simulink model "pi_seqOfVariableSizeIface"  (R2018b)
settings: Solver=FixedStepDiscrete  StartTime=0.0  StopTime=10.0  RelTol=1e-3
undefined symbols (not defined in the file): arr, nCount
settings Model: Creator=matlab  LastModifiedBy=matlab
settings DataIOCC: SaveOutput=off  SignalLogging=off  SaveTime=off
settings OptimizationCC: DefaultParameterBehavior=Inlined  EnhancedBackFolding=on  PassReuseOutputArgsAs=Individual arguments  OptimizeBlockOrder=speed  DifferentSizesBufferReuse=on  OptimizationCustomize=off
settings DebuggingCC: ParameterTunabilityLossMsg=error
settings SFSimCC: MATLABDynamicMemAlloc=off
settings RTWCC: SystemTargetFile=ert.tlc  TemplateMakefile=ert_default_tmf  PostCodeGenCommand=packNGo(buildInfo);  GenerateReport=on  IncludeHyperlinkInReport=on  LaunchReport=on  GenerateTraceInfo=on  GenerateTraceReport=on  GenerateTraceReportSl=on  GenerateTraceReportSf=on  GenerateTraceReportEml=on
settings CodeAppCC: ForceParamTrailComments=on  IgnoreCustomStorageClasses=off  OperatorAnnotations=on  SimulinkDataObjDesc=on  SFDataObjDesc=on  InsertBlockDesc=on
settings ERTTargetCC: TargetLangStandard=C99 (ISO)  GenerateSampleERTMain=on  InlinedParameterPlacement=NonHierarchical  ERTCustomFileTemplate=example_file_process.tlc

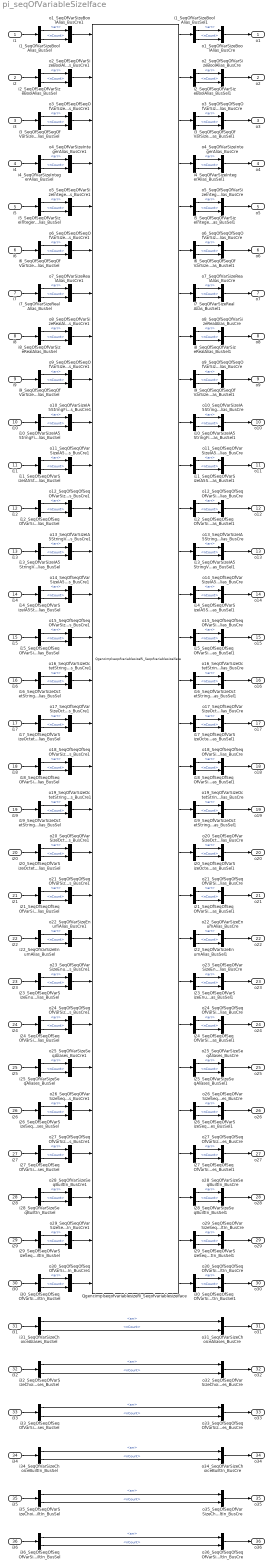
== system pi_seqOfVariableSizeIface ==
  i1 : Inport  OutDataTypeStr=Bus: SeqOfVarSizeBoolAlias  BusOutputAsStruct=on
  i2 : Inport  Port=2  OutDataTypeStr=Bus: SeqOfSeqOfVarSizeBoolAlias  BusOutputAsStruct=on
  i3 : Inport  Port=3  OutDataTypeStr=Bus: SeqOfSeqOfSeqOfVarSizeBoolAlias  BusOutputAsStruct=on
  i4 : Inport  Port=4  OutDataTypeStr=Bus: SeqOfVarSizeIntegerAlias  BusOutputAsStruct=on
  i5 : Inport  Port=5  OutDataTypeStr=Bus: SeqOfSeqOfVarSizeIntegerAlias  BusOutputAsStruct=on
  i6 : Inport  Port=6  OutDataTypeStr=Bus: SeqOfSeqOfSeqOfVarSizeIntegerAlias  BusOutputAsStruct=on
  i7 : Inport  Port=7  OutDataTypeStr=Bus: SeqOfVarSizeRealAlias  BusOutputAsStruct=on
  i8 : Inport  Port=8  OutDataTypeStr=Bus: SeqOfSeqOfVarSizeRealAlias  BusOutputAsStruct=on
  i9 : Inport  Port=9  OutDataTypeStr=Bus: SeqOfSeqOfSeqOfVarSizeRealAlias  BusOutputAsStruct=on
  i10 : Inport  Port=10  OutDataTypeStr=Bus: SeqOfVarSizeIA5StringFixedSizeAlias  BusOutputAsStruct=on
  i11 : Inport  Port=11  OutDataTypeStr=Bus: SeqOfSeqOfVarSizeIA5StringFixedSizeAlias  BusOutputAsStruct=on
  i12 : Inport  Port=12  OutDataTypeStr=Bus: SeqOfSeqOfSeqOfVarSizeIA5StringFixedSizeAlias  BusOutputAsStruct=on
  i13 : Inport  Port=13  OutDataTypeStr=Bus: SeqOfVarSizeIA5StringVarSizeAlias  BusOutputAsStruct=on
  i14 : Inport  Port=14  OutDataTypeStr=Bus: SeqOfSeqOfVarSizeIA5StringVarSizeAlias  BusOutputAsStruct=on
  i15 : Inport  Port=15  OutDataTypeStr=Bus: SeqOfSeqOfSeqOfVarSizeIA5StringVarSizeAlias  BusOutputAsStruct=on
  i16 : Inport  Port=16  OutDataTypeStr=Bus: SeqOfVarSizeOctetStringFixedSizeAlias  BusOutputAsStruct=on
  i17 : Inport  Port=17  OutDataTypeStr=Bus: SeqOfSeqOfVarSizeOctetStringFixedSizeAlias  BusOutputAsStruct=on
  i18 : Inport  Port=18  OutDataTypeStr=Bus: SeqOfSeqOfSeqOfVarSizeOctetStringFixedSizeAlias  BusOutputAsStruct=on
  i19 : Inport  Port=19  OutDataTypeStr=Bus: SeqOfVarSizeOctetStringVarSizeAlias  BusOutputAsStruct=on
  i20 : Inport  Port=20  OutDataTypeStr=Bus: SeqOfSeqOfVarSizeOctetStringVarSizeAlias  BusOutputAsStruct=on
  i21 : Inport  Port=21  OutDataTypeStr=Bus: SeqOfSeqOfSeqOfVarSizeOctetStringVarSizeAlias  BusOutputAsStruct=on
  i22 : Inport  Port=22  OutDataTypeStr=Bus: SeqOfVarSizeEnumAlias  BusOutputAsStruct=on
  i23 : Inport  Port=23  OutDataTypeStr=Bus: SeqOfSeqOfVarSizeEnumAlias  BusOutputAsStruct=on
  i24 : Inport  Port=24  OutDataTypeStr=Bus: SeqOfSeqOfSeqOfVarSizeEnumAlias  BusOutputAsStruct=on
  i25 : Inport  Port=25  OutDataTypeStr=Bus: SeqOfVarSizeSeqAliases  BusOutputAsStruct=on
  i26 : Inport  Port=26  OutDataTypeStr=Bus: SeqOfSeqOfVarSizeSeqAliases  BusOutputAsStruct=on
  i27 : Inport  Port=27  OutDataTypeStr=Bus: SeqOfSeqOfSeqOfVarSizeSeqAliases  BusOutputAsStruct=on
  i28 : Inport  Port=28  OutDataTypeStr=Bus: SeqOfVarSizeSeqBuiltIn  BusOutputAsStruct=on
  i29 : Inport  Port=29  OutDataTypeStr=Bus: SeqOfSeqOfVarSizeSeqBuiltIn  BusOutputAsStruct=on
  i30 : Inport  Port=30  OutDataTypeStr=Bus: SeqOfSeqOfSeqOfVarSizeSeqBuiltIn  BusOutputAsStruct=on
  i31 : Inport  Port=31  OutDataTypeStr=Bus: SeqOfVarSizeChoiceAliases  BusOutputAsStruct=on
  i32 : Inport  Port=32  OutDataTypeStr=Bus: SeqOfSeqOfVarSizeChoiceAliases  BusOutputAsStruct=on
  i33 : Inport  Port=33  OutDataTypeStr=Bus: SeqOfSeqOfSeqOfVarSizeChoiceAliases  BusOutputAsStruct=on
  i34 : Inport  Port=34  OutDataTypeStr=Bus: SeqOfVarSizeChoiceBuiltIn  BusOutputAsStruct=on
  i35 : Inport  Port=35  OutDataTypeStr=Bus: SeqOfSeqOfVarSizeChoiceBuiltIn  BusOutputAsStruct=on
  i36 : Inport  Port=36  OutDataTypeStr=Bus: SeqOfSeqOfSeqOfVarSizeChoiceBuiltIn  BusOutputAsStruct=on
  QgencimplseqofvariablesizeRi_Seqofvariablesizeiface : S-Function  FunctionName=QgencimplseqofvariablesizeRi_Seqofvariablesizeiface  SFunctionDeploymentMode=off  EnableBusSupport=off  mask(Legacy Function){SFunctionSpec=void qgencimplseqofvariablesize_RI_ri_seqOfVariableSizeIface(SeqOfVarSizeBoolAlias u1[1], SeqOfSeqOfVarSizeBoolAlias u2[1], SeqOfSeqOfSeqOfVarSizeBoolAlias u3[1], SeqOfVarSizeIntegerAlias u4[1], SeqOfSeqOfVarSizeIntegerAlias u5[1], SeqOfSeqOfSeqOfVarSizeIntegerAlias u6[1], SeqOfVarSizeRealAlias u7[1], SeqOfSeqOfVarSizeRealAlias u8[1], SeqOfSeqOfSeqOfVarSizeRealAlias u9[1], SeqOfVarSizeIA5StringFixedSizeAlias u10[1], SeqOfSeqOfVarSizeIA5StringFixedSizeAlias u11[1], SeqOfSeqOfSeqOfVarSizeIA5StringFixedSizeAlias u12[1], SeqOfVarSizeIA5StringVarSizeAlias u13[1], SeqOfSeqOfVarSizeIA5StringVarSizeAlias u14[1], SeqOfSeqOfSeqOfVarSizeIA5StringVarSizeAlias u15[1], SeqOfVarSizeOctetStringFixedSizeAlias u16[1], SeqOfSeqOfVarSizeOctetStringFixedSizeAlias u17[1], SeqOfSeqOfSeqOfVarSizeOctetStringFixedSizeAlias u18[1], SeqOfVarSizeOctetStringVarSizeAlias u19[1], SeqOfSeqOfVarSizeOctetStringVarSizeAlias u20[1], SeqOfSeqOfSeqOfVarSizeOctetStringVarSizeAlias u21[1], SeqOfVarSizeEnumAlias u22[1], SeqOfSeqOfVarSizeEnumAlias u23[1], SeqOfSeqOfSeqOfVarSizeEnumAlias u24[1], SeqOfVarSizeSeqAliases u25[1], SeqOfSeqOfVarSizeSeqAliases u26[1], SeqOfSeqOfSeqOfVarSizeSeqAliases u27[1], SeqOfVarSizeSeqBuiltIn u28[1], SeqOfSeqOfVarSizeSeqBuiltIn u29[1], SeqOfSeqOfSeqOfVarSizeSeqBuiltIn u30[1], SeqOfVarSizeBoolAlias y1[1], SeqOfSeqOfVarSizeBoolAlias y2[1], SeqOfSeqOfSeqOfVarSizeBoolAlias y3[1], SeqOfVarSizeIntegerAlias y4[1], SeqOfSeqOfVarSizeIntegerAlias y5[1], SeqOfSeqOfSeqOfVarSizeIntegerAlias y6[1], SeqOfVarSizeRealAlias y7[1], SeqOfSeqOfVarSizeRealAlias y8[1], SeqOfSeqOfSeqOfVarSizeRealAlias y9[1], SeqOfVarSizeIA5StringFixedSizeAlias y10[1], SeqOfSeqOfVarSizeIA5StringFixedSizeAlias y11[1], SeqOfSeqOfSeqOfVarSizeIA5StringFixedSizeAlias y12[1], SeqOfVarSizeIA5StringVarSizeAlias y13[1], SeqOfSeqOfVarSizeIA5StringVarSizeAlias y14[1], SeqOfSeqOfSeqOfVarSizeIA5StringVarSizeAlias y15[1], SeqOfVarSizeOctetStringFixedSizeAlias y16[1], SeqOfSeqOfVarSizeOctetStringFixedSizeAlias y17[1], SeqOfSeqOfSeqOfVarSizeOctetStringFixedSizeAlias y18[1], SeqOfVarSizeOctetStringVarSizeAlias y19[1], SeqOfSeqOfVarSizeOctetStringVarSizeAlias y20[1], SeqOfSeqOfSeqOfVarSizeOctetStringVarSizeAlias y21[1], SeqOfVarSizeEnumAlias y22[1], SeqOfSeqOfVarSizeEnumAlias y23[1], SeqOfSeqOfSeqOfVarSizeEnumAlias y24[1], SeqOfVarSizeSeqAliases y25[1], SeqOfSeqOfVarSizeSeqAliases y26[1], SeqOfSeqOfSeqOfVarSizeSeqAliases y27[1], SeqOfVarSizeSeqBuiltIn y28[1], SeqOfSeqOfVarSizeSeqBuiltIn y29[1], SeqOfSeqOfSeqOfVarSizeSeqBuiltIn y30[1]), ShowSpec=off}
      mask prompts: ShowSpec "Display function specification"
      mask help:
      | This block allows you to call the legacy functions specified by the following Legacy Code Tool definition:
      | def.SFunctionName = 'QgencimplseqofvariablesizeRi_Seqofvariablesizeiface';
      | def.OutputFcnSpec = 'void qgencimplseqofvariablesize_RI_ri_seqOfVariableSizeIface(SeqOfVarSizeBoolAlias u1[1], SeqOfSeqOfVarSizeBoolAlias u2[1], SeqOfSeqOfSeqOfVarSizeBoolAlias u3[1], SeqOfVarSizeIntegerAlias u4[1], SeqOfSeqOfVarSizeIntegerAlias u5[1], SeqOfSeqOfSeqOfVarSizeIntegerAlias u6[1], SeqOfVarSizeRealAlias u7[1], SeqOfSeqOfVarSizeRealAlias u8[1], SeqOfSeqOfSeqOfVarSizeRealAlias u9[1], SeqOfVarSizeIA5StringFixedSizeAlias u10[1], SeqOfSeqOfVarSizeIA5StringFixedSizeAlias u11[1], SeqOfSeqOfSeqOfVarSizeIA5StringFixedSizeAlias u12[1], SeqOfVarSizeIA5StringVarSizeAlias u13[1], SeqOfSeqOfVarSizeIA5StringVarSizeAlias u14[1], SeqOfSeqOfSeqOfVarSizeIA5StringVarSizeAlias u15[1], SeqOfVarSizeOctetStringFixedSizeAlias u16[1], SeqOfSeqOfVarSizeOctetStringFixedSizeAlias u17[1], SeqOfSeqOfSeqOfVarSizeOctetStringFixedSizeAlias u18[1], SeqOfVarSizeOctetStringVarSizeAlias u19[1], SeqOfSeqOfVarSizeOctetStringVarSizeAlias u20[1], SeqOfSeqOfSeqOfVarSizeOctetStringVarSizeAlias u21[1], SeqOfVarSizeEnumAlias u22[1], SeqOfSeqOfVarSizeEnumAlias u23[1], SeqOfSeqOfSeqOfVarSizeEnumAlias u24[1], SeqOfVarSizeSeqAliases u25[1], SeqOfSeqOfVarSizeSeqAliases u26[1], SeqOfSeqOfSeqOfVarSizeSeqAliases u27[1], SeqOfVarSizeSeqBuiltIn u28[1], SeqOfSeqOfVarSizeSeqBuiltIn u29[1], SeqOfSeqOfSeqOfVarSizeSeqBuiltIn u30[1], SeqOfVarSizeBoolAlias y1[1], SeqOfSeqOfVarSizeBoolAlias y2[1], SeqOfSeqOfSeqOfVarSizeBoolAlias y3[1], SeqOfVarSizeIntegerAlias y4[1], SeqOfSeqOfVarSizeIntegerAlias y5[1], SeqOfSeqOfSeqOfVarSizeIntegerAlias y6[1], SeqOfVarSizeRealAlias y7[1], SeqOfSeqOfVarSizeRealAlias y8[1], SeqOfSeqOfSeqOfVarSizeRealAlias y9[1], SeqOfVarSizeIA5StringFixedSizeAlias y10[1], SeqOfSeqOfVarSizeIA5StringFixedSizeAlias y11[1], SeqOfSeqOfSeqOfVarSizeIA5StringFixedSizeAlias y12[1], SeqOfVarSizeIA5StringVarSizeAlias y13[1], SeqOfSeqOfVarSizeIA5StringVarSizeAlias y14[1], SeqOfSeqOfSeqOfVarSizeIA5StringVarSizeAlias y15[1], SeqOfVarSizeOctetStringFixedSizeAlias y16[1], SeqOfSeqOfVarSizeOctetStringFixedSizeAlias y17[1], SeqOfSeqOfSeqOfVarSizeOctetStringFixedSizeAlias y18[1], SeqOfVarSizeOctetStringVarSizeAlias y19[1], SeqOfSeqOfVarSizeOctetStringVarSizeAlias y20[1], SeqOfSeqOfSeqOfVarSizeOctetStringVarSizeAlias y21[1], SeqOfVarSizeEnumAlias y22[1], SeqOfSeqOfVarSizeEnumAlias y23[1], SeqOfSeqOfSeqOfVarSizeEnumAlias y24[1], SeqOfVarSizeSeqAliases y25[1], SeqOfSeqOfVarSizeSeqAliases y26[1], SeqOfSeqOfSeqOfVarSizeSeqAliases y27[1], SeqOfVarSizeSeqBuiltIn y28[1], SeqOfSeqOfVarSizeSeqBuiltIn y29[1], SeqOfSeqOfSeqOfVarSizeSeqBuiltIn y30[1])';
      | def.HeaderFiles = {'qgencimplseqofvariablesize_invoke_ri.h'};
      | def.SourceFiles = {'qgencimplseqofvariablesize_invoke_ri.c'};
      | def.IncPaths = {'..\..\..\dataview\C'};
      mask Help: <p>This block was generated automatically by the Legacy Code Tool. For detailed help on this tool, call<a href="matlab:legacy_code('help')"> legacy_code('help')</a>.</p>
      mask Callback ShowSpec:
      | if strcmp(get_param(gcbh, 'ShowSpec'), 'on')
      |   set_param(gcbh, 'MaskDisplay', sprintf('fprintf(''%s'');', get_param(gcbh, 'SFunctionSpec')));
      | else
      |   set_param(gcbh, 'MaskDisplay', sprintf('fprintf(''%s'');', get_param(gcbh, 'FunctionName')));
      | end
      mask Display: fprintf('QgencimplseqofvariablesizeRi_Seqofvariablesizeiface');
  i10_SeqOfVarSizeIA5StringFixedSizeAlias_BusSel : BusSelector  OutputSignals=arr,nCount
  i10_SeqOfVarSizeIA5StringFixedSizeAlias_BusSel1 : BusSelector  OutputSignals=arr,nCount
  i11_SeqOfSeqOfVarSizeIA5StringFixedSizeAlias_BusSel : BusSelector  OutputSignals=arr,nCount
  i11_SeqOfSeqOfVarSizeIA5StringFixedSizeAlias_BusSel1 : BusSelector  OutputSignals=arr,nCount
  i12_SeqOfSeqOfSeqOfVarSizeIA5StringFixedSizeAlias_BusSel : BusSelector  OutputSignals=arr,nCount
  i12_SeqOfSeqOfSeqOfVarSizeIA5StringFixedSizeAlias_BusSel1 : BusSelector  OutputSignals=arr,nCount
  i13_SeqOfVarSizeIA5StringVarSizeAlias_BusSel : BusSelector  OutputSignals=arr,nCount
  i13_SeqOfVarSizeIA5StringVarSizeAlias_BusSel1 : BusSelector  OutputSignals=arr,nCount
  i14_SeqOfSeqOfVarSizeIA5StringVarSizeAlias_BusSel : BusSelector  OutputSignals=arr,nCount
  i14_SeqOfSeqOfVarSizeIA5StringVarSizeAlias_BusSel1 : BusSelector  OutputSignals=arr,nCount
  i15_SeqOfSeqOfSeqOfVarSizeIA5StringVarSizeAlias_BusSel : BusSelector  OutputSignals=arr,nCount
  i15_SeqOfSeqOfSeqOfVarSizeIA5StringVarSizeAlias_BusSel1 : BusSelector  OutputSignals=arr,nCount
  i16_SeqOfVarSizeOctetStringFixedSizeAlias_BusSel : BusSelector  OutputSignals=arr,nCount
  i16_SeqOfVarSizeOctetStringFixedSizeAlias_BusSel1 : BusSelector  OutputSignals=arr,nCount
  i17_SeqOfSeqOfVarSizeOctetStringFixedSizeAlias_BusSel : BusSelector  OutputSignals=arr,nCount
  i17_SeqOfSeqOfVarSizeOctetStringFixedSizeAlias_BusSel1 : BusSelector  OutputSignals=arr,nCount
  i18_SeqOfSeqOfSeqOfVarSizeOctetStringFixedSizeAlias_BusSel : BusSelector  OutputSignals=arr,nCount
  i18_SeqOfSeqOfSeqOfVarSizeOctetStringFixedSizeAlias_BusSel1 : BusSelector  OutputSignals=arr,nCount
  i19_SeqOfVarSizeOctetStringVarSizeAlias_BusSel : BusSelector  OutputSignals=arr,nCount
  i19_SeqOfVarSizeOctetStringVarSizeAlias_BusSel1 : BusSelector  OutputSignals=arr,nCount
  i1_SeqOfVarSizeBoolAlias_BusSel : BusSelector  OutputSignals=arr,nCount
  i1_SeqOfVarSizeBoolAlias_BusSel1 : BusSelector  OutputSignals=arr,nCount
  i20_SeqOfSeqOfVarSizeOctetStringVarSizeAlias_BusSel : BusSelector  OutputSignals=arr,nCount
  i20_SeqOfSeqOfVarSizeOctetStringVarSizeAlias_BusSel1 : BusSelector  OutputSignals=arr,nCount
  i21_SeqOfSeqOfSeqOfVarSizeOctetStringVarSizeAlias_BusSel : BusSelector  OutputSignals=arr,nCount
  i21_SeqOfSeqOfSeqOfVarSizeOctetStringVarSizeAlias_BusSel1 : BusSelector  OutputSignals=arr,nCount
  i22_SeqOfVarSizeEnumAlias_BusSel : BusSelector  OutputSignals=arr,nCount
  i22_SeqOfVarSizeEnumAlias_BusSel1 : BusSelector  OutputSignals=arr,nCount
  i23_SeqOfSeqOfVarSizeEnumAlias_BusSel : BusSelector  OutputSignals=arr,nCount
  i23_SeqOfSeqOfVarSizeEnumAlias_BusSel1 : BusSelector  OutputSignals=arr,nCount
  i24_SeqOfSeqOfSeqOfVarSizeEnumAlias_BusSel : BusSelector  OutputSignals=arr,nCount
  i24_SeqOfSeqOfSeqOfVarSizeEnumAlias_BusSel1 : BusSelector  OutputSignals=arr,nCount
  i25_SeqOfVarSizeSeqAliases_BusSel : BusSelector  OutputSignals=arr,nCount
  i25_SeqOfVarSizeSeqAliases_BusSel1 : BusSelector  OutputSignals=arr,nCount
  i26_SeqOfSeqOfVarSizeSeqAliases_BusSel : BusSelector  OutputSignals=arr,nCount
  i26_SeqOfSeqOfVarSizeSeqAliases_BusSel1 : BusSelector  OutputSignals=arr,nCount
  i27_SeqOfSeqOfSeqOfVarSizeSeqAliases_BusSel : BusSelector  OutputSignals=arr,nCount
  i27_SeqOfSeqOfSeqOfVarSizeSeqAliases_BusSel1 : BusSelector  OutputSignals=arr,nCount
  i28_SeqOfVarSizeSeqBuiltIn_BusSel : BusSelector  OutputSignals=arr,nCount
  i28_SeqOfVarSizeSeqBuiltIn_BusSel1 : BusSelector  OutputSignals=arr,nCount
  i29_SeqOfSeqOfVarSizeSeqBuiltIn_BusSel : BusSelector  OutputSignals=arr,nCount
  i29_SeqOfSeqOfVarSizeSeqBuiltIn_BusSel1 : BusSelector  OutputSignals=arr,nCount
  i2_SeqOfSeqOfVarSizeBoolAlias_BusSel : BusSelector  OutputSignals=arr,nCount
  i2_SeqOfSeqOfVarSizeBoolAlias_BusSel1 : BusSelector  OutputSignals=arr,nCount
  i30_SeqOfSeqOfSeqOfVarSizeSeqBuiltIn_BusSel : BusSelector  OutputSignals=arr,nCount
  i30_SeqOfSeqOfSeqOfVarSizeSeqBuiltIn_BusSel1 : BusSelector  OutputSignals=arr,nCount
  i31_SeqOfVarSizeChoiceAliases_BusSel : BusSelector  OutputSignals=arr,nCount
  i32_SeqOfSeqOfVarSizeChoiceAliases_BusSel : BusSelector  OutputSignals=arr,nCount
  i33_SeqOfSeqOfSeqOfVarSizeChoiceAliases_BusSel : BusSelector  OutputSignals=arr,nCount
  i34_SeqOfVarSizeChoiceBuiltIn_BusSel : BusSelector  OutputSignals=arr,nCount
  i35_SeqOfSeqOfVarSizeChoiceBuiltIn_BusSel : BusSelector  OutputSignals=arr,nCount
  i36_SeqOfSeqOfSeqOfVarSizeChoiceBuiltIn_BusSel : BusSelector  OutputSignals=arr,nCount
  i3_SeqOfSeqOfSeqOfVarSizeBoolAlias_BusSel : BusSelector  OutputSignals=arr,nCount
  i3_SeqOfSeqOfSeqOfVarSizeBoolAlias_BusSel1 : BusSelector  OutputSignals=arr,nCount
  i4_SeqOfVarSizeIntegerAlias_BusSel : BusSelector  OutputSignals=arr,nCount
  i4_SeqOfVarSizeIntegerAlias_BusSel1 : BusSelector  OutputSignals=arr,nCount
  i5_SeqOfSeqOfVarSizeIntegerAlias_BusSel : BusSelector  OutputSignals=arr,nCount
  i5_SeqOfSeqOfVarSizeIntegerAlias_BusSel1 : BusSelector  OutputSignals=arr,nCount
  i6_SeqOfSeqOfSeqOfVarSizeIntegerAlias_BusSel : BusSelector  OutputSignals=arr,nCount
  i6_SeqOfSeqOfSeqOfVarSizeIntegerAlias_BusSel1 : BusSelector  OutputSignals=arr,nCount
  i7_SeqOfVarSizeRealAlias_BusSel : BusSelector  OutputSignals=arr,nCount
  i7_SeqOfVarSizeRealAlias_BusSel1 : BusSelector  OutputSignals=arr,nCount
  i8_SeqOfSeqOfVarSizeRealAlias_BusSel : BusSelector  OutputSignals=arr,nCount
  i8_SeqOfSeqOfVarSizeRealAlias_BusSel1 : BusSelector  OutputSignals=arr,nCount
  i9_SeqOfSeqOfSeqOfVarSizeRealAlias_BusSel : BusSelector  OutputSignals=arr,nCount
  i9_SeqOfSeqOfSeqOfVarSizeRealAlias_BusSel1 : BusSelector  OutputSignals=arr,nCount
  o10_SeqOfVarSizeIA5StringFixedSizeAlias_BusCre : BusCreator  Inputs=arr,nCount  OutDataTypeStr=Bus: SeqOfVarSizeIA5StringFixedSizeAlias  NonVirtualBus=on
  o10_SeqOfVarSizeIA5StringFixedSizeAlias_BusCre1 : BusCreator  Inputs=arr,nCount  OutDataTypeStr=Bus: SeqOfVarSizeIA5StringFixedSizeAlias  NonVirtualBus=on
  o11_SeqOfSeqOfVarSizeIA5StringFixedSizeAlias_BusCre : BusCreator  Inputs=arr,nCount  OutDataTypeStr=Bus: SeqOfSeqOfVarSizeIA5StringFixedSizeAlias  NonVirtualBus=on
  o11_SeqOfSeqOfVarSizeIA5StringFixedSizeAlias_BusCre1 : BusCreator  Inputs=arr,nCount  OutDataTypeStr=Bus: SeqOfSeqOfVarSizeIA5StringFixedSizeAlias  NonVirtualBus=on
  o12_SeqOfSeqOfSeqOfVarSizeIA5StringFixedSizeAlias_BusCre : BusCreator  Inputs=arr,nCount  OutDataTypeStr=Bus: SeqOfSeqOfSeqOfVarSizeIA5StringFixedSizeAlias  NonVirtualBus=on
  o12_SeqOfSeqOfSeqOfVarSizeIA5StringFixedSizeAlias_BusCre1 : BusCreator  Inputs=arr,nCount  OutDataTypeStr=Bus: SeqOfSeqOfSeqOfVarSizeIA5StringFixedSizeAlias  NonVirtualBus=on
  o13_SeqOfVarSizeIA5StringVarSizeAlias_BusCre : BusCreator  Inputs=arr,nCount  OutDataTypeStr=Bus: SeqOfVarSizeIA5StringVarSizeAlias  NonVirtualBus=on
  o13_SeqOfVarSizeIA5StringVarSizeAlias_BusCre1 : BusCreator  Inputs=arr,nCount  OutDataTypeStr=Bus: SeqOfVarSizeIA5StringVarSizeAlias  NonVirtualBus=on
  o14_SeqOfSeqOfVarSizeIA5StringVarSizeAlias_BusCre : BusCreator  Inputs=arr,nCount  OutDataTypeStr=Bus: SeqOfSeqOfVarSizeIA5StringVarSizeAlias  NonVirtualBus=on
  o14_SeqOfSeqOfVarSizeIA5StringVarSizeAlias_BusCre1 : BusCreator  Inputs=arr,nCount  OutDataTypeStr=Bus: SeqOfSeqOfVarSizeIA5StringVarSizeAlias  NonVirtualBus=on
  o15_SeqOfSeqOfSeqOfVarSizeIA5StringVarSizeAlias_BusCre : BusCreator  Inputs=arr,nCount  OutDataTypeStr=Bus: SeqOfSeqOfSeqOfVarSizeIA5StringVarSizeAlias  NonVirtualBus=on
  o15_SeqOfSeqOfSeqOfVarSizeIA5StringVarSizeAlias_BusCre1 : BusCreator  Inputs=arr,nCount  OutDataTypeStr=Bus: SeqOfSeqOfSeqOfVarSizeIA5StringVarSizeAlias  NonVirtualBus=on
  o16_SeqOfVarSizeOctetStringFixedSizeAlias_BusCre : BusCreator  Inputs=arr,nCount  OutDataTypeStr=Bus: SeqOfVarSizeOctetStringFixedSizeAlias  NonVirtualBus=on
  o16_SeqOfVarSizeOctetStringFixedSizeAlias_BusCre1 : BusCreator  Inputs=arr,nCount  OutDataTypeStr=Bus: SeqOfVarSizeOctetStringFixedSizeAlias  NonVirtualBus=on
  o17_SeqOfSeqOfVarSizeOctetStringFixedSizeAlias_BusCre : BusCreator  Inputs=arr,nCount  OutDataTypeStr=Bus: SeqOfSeqOfVarSizeOctetStringFixedSizeAlias  NonVirtualBus=on
  o17_SeqOfSeqOfVarSizeOctetStringFixedSizeAlias_BusCre1 : BusCreator  Inputs=arr,nCount  OutDataTypeStr=Bus: SeqOfSeqOfVarSizeOctetStringFixedSizeAlias  NonVirtualBus=on
  o18_SeqOfSeqOfSeqOfVarSizeOctetStringFixedSizeAlias_BusCre : BusCreator  Inputs=arr,nCount  OutDataTypeStr=Bus: SeqOfSeqOfSeqOfVarSizeOctetStringFixedSizeAlias  NonVirtualBus=on
  o18_SeqOfSeqOfSeqOfVarSizeOctetStringFixedSizeAlias_BusCre1 : BusCreator  Inputs=arr,nCount  OutDataTypeStr=Bus: SeqOfSeqOfSeqOfVarSizeOctetStringFixedSizeAlias  NonVirtualBus=on
  o19_SeqOfVarSizeOctetStringVarSizeAlias_BusCre : BusCreator  Inputs=arr,nCount  OutDataTypeStr=Bus: SeqOfVarSizeOctetStringVarSizeAlias  NonVirtualBus=on
  o19_SeqOfVarSizeOctetStringVarSizeAlias_BusCre1 : BusCreator  Inputs=arr,nCount  OutDataTypeStr=Bus: SeqOfVarSizeOctetStringVarSizeAlias  NonVirtualBus=on
  o1_SeqOfVarSizeBoolAlias_BusCre : BusCreator  Inputs=arr,nCount  OutDataTypeStr=Bus: SeqOfVarSizeBoolAlias  NonVirtualBus=on
  o1_SeqOfVarSizeBoolAlias_BusCre1 : BusCreator  Inputs=arr,nCount  OutDataTypeStr=Bus: SeqOfVarSizeBoolAlias  NonVirtualBus=on
  o20_SeqOfSeqOfVarSizeOctetStringVarSizeAlias_BusCre : BusCreator  Inputs=arr,nCount  OutDataTypeStr=Bus: SeqOfSeqOfVarSizeOctetStringVarSizeAlias  NonVirtualBus=on
  o20_SeqOfSeqOfVarSizeOctetStringVarSizeAlias_BusCre1 : BusCreator  Inputs=arr,nCount  OutDataTypeStr=Bus: SeqOfSeqOfVarSizeOctetStringVarSizeAlias  NonVirtualBus=on
  o21_SeqOfSeqOfSeqOfVarSizeOctetStringVarSizeAlias_BusCre : BusCreator  Inputs=arr,nCount  OutDataTypeStr=Bus: SeqOfSeqOfSeqOfVarSizeOctetStringVarSizeAlias  NonVirtualBus=on
  o21_SeqOfSeqOfSeqOfVarSizeOctetStringVarSizeAlias_BusCre1 : BusCreator  Inputs=arr,nCount  OutDataTypeStr=Bus: SeqOfSeqOfSeqOfVarSizeOctetStringVarSizeAlias  NonVirtualBus=on
  o22_SeqOfVarSizeEnumAlias_BusCre : BusCreator  Inputs=arr,nCount  OutDataTypeStr=Bus: SeqOfVarSizeEnumAlias  NonVirtualBus=on
  o22_SeqOfVarSizeEnumAlias_BusCre1 : BusCreator  Inputs=arr,nCount  OutDataTypeStr=Bus: SeqOfVarSizeEnumAlias  NonVirtualBus=on
  o23_SeqOfSeqOfVarSizeEnumAlias_BusCre : BusCreator  Inputs=arr,nCount  OutDataTypeStr=Bus: SeqOfSeqOfVarSizeEnumAlias  NonVirtualBus=on
  o23_SeqOfSeqOfVarSizeEnumAlias_BusCre1 : BusCreator  Inputs=arr,nCount  OutDataTypeStr=Bus: SeqOfSeqOfVarSizeEnumAlias  NonVirtualBus=on
  o24_SeqOfSeqOfSeqOfVarSizeEnumAlias_BusCre : BusCreator  Inputs=arr,nCount  OutDataTypeStr=Bus: SeqOfSeqOfSeqOfVarSizeEnumAlias  NonVirtualBus=on
  o24_SeqOfSeqOfSeqOfVarSizeEnumAlias_BusCre1 : BusCreator  Inputs=arr,nCount  OutDataTypeStr=Bus: SeqOfSeqOfSeqOfVarSizeEnumAlias  NonVirtualBus=on
  o25_SeqOfVarSizeSeqAliases_BusCre : BusCreator  Inputs=arr,nCount  OutDataTypeStr=Bus: SeqOfVarSizeSeqAliases  NonVirtualBus=on
  o25_SeqOfVarSizeSeqAliases_BusCre1 : BusCreator  Inputs=arr,nCount  OutDataTypeStr=Bus: SeqOfVarSizeSeqAliases  NonVirtualBus=on
  o26_SeqOfSeqOfVarSizeSeqAliases_BusCre : BusCreator  Inputs=arr,nCount  OutDataTypeStr=Bus: SeqOfSeqOfVarSizeSeqAliases  NonVirtualBus=on
  o26_SeqOfSeqOfVarSizeSeqAliases_BusCre1 : BusCreator  Inputs=arr,nCount  OutDataTypeStr=Bus: SeqOfSeqOfVarSizeSeqAliases  NonVirtualBus=on
  o27_SeqOfSeqOfSeqOfVarSizeSeqAliases_BusCre : BusCreator  Inputs=arr,nCount  OutDataTypeStr=Bus: SeqOfSeqOfSeqOfVarSizeSeqAliases  NonVirtualBus=on
  o27_SeqOfSeqOfSeqOfVarSizeSeqAliases_BusCre1 : BusCreator  Inputs=arr,nCount  OutDataTypeStr=Bus: SeqOfSeqOfSeqOfVarSizeSeqAliases  NonVirtualBus=on
  o28_SeqOfVarSizeSeqBuiltIn_BusCre : BusCreator  Inputs=arr,nCount  OutDataTypeStr=Bus: SeqOfVarSizeSeqBuiltIn  NonVirtualBus=on
  o28_SeqOfVarSizeSeqBuiltIn_BusCre1 : BusCreator  Inputs=arr,nCount  OutDataTypeStr=Bus: SeqOfVarSizeSeqBuiltIn  NonVirtualBus=on
  o29_SeqOfSeqOfVarSizeSeqBuiltIn_BusCre : BusCreator  Inputs=arr,nCount  OutDataTypeStr=Bus: SeqOfSeqOfVarSizeSeqBuiltIn  NonVirtualBus=on
  o29_SeqOfSeqOfVarSizeSeqBuiltIn_BusCre1 : BusCreator  Inputs=arr,nCount  OutDataTypeStr=Bus: SeqOfSeqOfVarSizeSeqBuiltIn  NonVirtualBus=on
  o2_SeqOfSeqOfVarSizeBoolAlias_BusCre : BusCreator  Inputs=arr,nCount  OutDataTypeStr=Bus: SeqOfSeqOfVarSizeBoolAlias  NonVirtualBus=on
  o2_SeqOfSeqOfVarSizeBoolAlias_BusCre1 : BusCreator  Inputs=arr,nCount  OutDataTypeStr=Bus: SeqOfSeqOfVarSizeBoolAlias  NonVirtualBus=on
  o30_SeqOfSeqOfSeqOfVarSizeSeqBuiltIn_BusCre : BusCreator  Inputs=arr,nCount  OutDataTypeStr=Bus: SeqOfSeqOfSeqOfVarSizeSeqBuiltIn  NonVirtualBus=on
  o30_SeqOfSeqOfSeqOfVarSizeSeqBuiltIn_BusCre1 : BusCreator  Inputs=arr,nCount  OutDataTypeStr=Bus: SeqOfSeqOfSeqOfVarSizeSeqBuiltIn  NonVirtualBus=on
  o31_SeqOfVarSizeChoiceAliases_BusCre : BusCreator  Inputs=arr,nCount  OutDataTypeStr=Bus: SeqOfVarSizeChoiceAliases  NonVirtualBus=on
  o32_SeqOfSeqOfVarSizeChoiceAliases_BusCre : BusCreator  Inputs=arr,nCount  OutDataTypeStr=Bus: SeqOfSeqOfVarSizeChoiceAliases  NonVirtualBus=on
  o33_SeqOfSeqOfSeqOfVarSizeChoiceAliases_BusCre : BusCreator  Inputs=arr,nCount  OutDataTypeStr=Bus: SeqOfSeqOfSeqOfVarSizeChoiceAliases  NonVirtualBus=on
  o34_SeqOfVarSizeChoiceBuiltIn_BusCre : BusCreator  Inputs=arr,nCount  OutDataTypeStr=Bus: SeqOfVarSizeChoiceBuiltIn  NonVirtualBus=on
  o35_SeqOfSeqOfVarSizeChoiceBuiltIn_BusCre : BusCreator  Inputs=arr,nCount  OutDataTypeStr=Bus: SeqOfSeqOfVarSizeChoiceBuiltIn  NonVirtualBus=on
  o36_SeqOfSeqOfSeqOfVarSizeChoiceBuiltIn_BusCre : BusCreator  Inputs=arr,nCount  OutDataTypeStr=Bus: SeqOfSeqOfSeqOfVarSizeChoiceBuiltIn  NonVirtualBus=on
  o3_SeqOfSeqOfSeqOfVarSizeBoolAlias_BusCre : BusCreator  Inputs=arr,nCount  OutDataTypeStr=Bus: SeqOfSeqOfSeqOfVarSizeBoolAlias  NonVirtualBus=on
  o3_SeqOfSeqOfSeqOfVarSizeBoolAlias_BusCre1 : BusCreator  Inputs=arr,nCount  OutDataTypeStr=Bus: SeqOfSeqOfSeqOfVarSizeBoolAlias  NonVirtualBus=on
  o4_SeqOfVarSizeIntegerAlias_BusCre : BusCreator  Inputs=arr,nCount  OutDataTypeStr=Bus: SeqOfVarSizeIntegerAlias  NonVirtualBus=on
  o4_SeqOfVarSizeIntegerAlias_BusCre1 : BusCreator  Inputs=arr,nCount  OutDataTypeStr=Bus: SeqOfVarSizeIntegerAlias  NonVirtualBus=on
  o5_SeqOfSeqOfVarSizeIntegerAlias_BusCre : BusCreator  Inputs=arr,nCount  OutDataTypeStr=Bus: SeqOfSeqOfVarSizeIntegerAlias  NonVirtualBus=on
  o5_SeqOfSeqOfVarSizeIntegerAlias_BusCre1 : BusCreator  Inputs=arr,nCount  OutDataTypeStr=Bus: SeqOfSeqOfVarSizeIntegerAlias  NonVirtualBus=on
  o6_SeqOfSeqOfSeqOfVarSizeIntegerAlias_BusCre : BusCreator  Inputs=arr,nCount  OutDataTypeStr=Bus: SeqOfSeqOfSeqOfVarSizeIntegerAlias  NonVirtualBus=on
  o6_SeqOfSeqOfSeqOfVarSizeIntegerAlias_BusCre1 : BusCreator  Inputs=arr,nCount  OutDataTypeStr=Bus: SeqOfSeqOfSeqOfVarSizeIntegerAlias  NonVirtualBus=on
  o7_SeqOfVarSizeRealAlias_BusCre : BusCreator  Inputs=arr,nCount  OutDataTypeStr=Bus: SeqOfVarSizeRealAlias  NonVirtualBus=on
  o7_SeqOfVarSizeRealAlias_BusCre1 : BusCreator  Inputs=arr,nCount  OutDataTypeStr=Bus: SeqOfVarSizeRealAlias  NonVirtualBus=on
  o8_SeqOfSeqOfVarSizeRealAlias_BusCre : BusCreator  Inputs=arr,nCount  OutDataTypeStr=Bus: SeqOfSeqOfVarSizeRealAlias  NonVirtualBus=on
  o8_SeqOfSeqOfVarSizeRealAlias_BusCre1 : BusCreator  Inputs=arr,nCount  OutDataTypeStr=Bus: SeqOfSeqOfVarSizeRealAlias  NonVirtualBus=on
  o9_SeqOfSeqOfSeqOfVarSizeRealAlias_BusCre : BusCreator  Inputs=arr,nCount  OutDataTypeStr=Bus: SeqOfSeqOfSeqOfVarSizeRealAlias  NonVirtualBus=on
  o9_SeqOfSeqOfSeqOfVarSizeRealAlias_BusCre1 : BusCreator  Inputs=arr,nCount  OutDataTypeStr=Bus: SeqOfSeqOfSeqOfVarSizeRealAlias  NonVirtualBus=on
  o1 : Outport  OutDataTypeStr=Bus: SeqOfVarSizeBoolAlias  BusOutputAsStruct=on
  o2 : Outport  Port=2  OutDataTypeStr=Bus: SeqOfSeqOfVarSizeBoolAlias  BusOutputAsStruct=on
  o3 : Outport  Port=3  OutDataTypeStr=Bus: SeqOfSeqOfSeqOfVarSizeBoolAlias  BusOutputAsStruct=on
  o4 : Outport  Port=4  OutDataTypeStr=Bus: SeqOfVarSizeIntegerAlias  BusOutputAsStruct=on
  o5 : Outport  Port=5  OutDataTypeStr=Bus: SeqOfSeqOfVarSizeIntegerAlias  BusOutputAsStruct=on
  o6 : Outport  Port=6  OutDataTypeStr=Bus: SeqOfSeqOfSeqOfVarSizeIntegerAlias  BusOutputAsStruct=on
  o7 : Outport  Port=7  OutDataTypeStr=Bus: SeqOfVarSizeRealAlias  BusOutputAsStruct=on
  o8 : Outport  Port=8  OutDataTypeStr=Bus: SeqOfSeqOfVarSizeRealAlias  BusOutputAsStruct=on
  o9 : Outport  Port=9  OutDataTypeStr=Bus: SeqOfSeqOfSeqOfVarSizeRealAlias  BusOutputAsStruct=on
  o10 : Outport  Port=10  OutDataTypeStr=Bus: SeqOfVarSizeIA5StringFixedSizeAlias  BusOutputAsStruct=on
  o11 : Outport  Port=11  OutDataTypeStr=Bus: SeqOfSeqOfVarSizeIA5StringFixedSizeAlias  BusOutputAsStruct=on
  o12 : Outport  Port=12  OutDataTypeStr=Bus: SeqOfSeqOfSeqOfVarSizeIA5StringFixedSizeAlias  BusOutputAsStruct=on
  o13 : Outport  Port=13  OutDataTypeStr=Bus: SeqOfVarSizeIA5StringVarSizeAlias  BusOutputAsStruct=on
  o14 : Outport  Port=14  OutDataTypeStr=Bus: SeqOfSeqOfVarSizeIA5StringVarSizeAlias  BusOutputAsStruct=on
  o15 : Outport  Port=15  OutDataTypeStr=Bus: SeqOfSeqOfSeqOfVarSizeIA5StringVarSizeAlias  BusOutputAsStruct=on
  o16 : Outport  Port=16  OutDataTypeStr=Bus: SeqOfVarSizeOctetStringFixedSizeAlias  BusOutputAsStruct=on
  o17 : Outport  Port=17  OutDataTypeStr=Bus: SeqOfSeqOfVarSizeOctetStringFixedSizeAlias  BusOutputAsStruct=on
  o18 : Outport  Port=18  OutDataTypeStr=Bus: SeqOfSeqOfSeqOfVarSizeOctetStringFixedSizeAlias  BusOutputAsStruct=on
  o19 : Outport  Port=19  OutDataTypeStr=Bus: SeqOfVarSizeOctetStringVarSizeAlias  BusOutputAsStruct=on
  o20 : Outport  Port=20  OutDataTypeStr=Bus: SeqOfSeqOfVarSizeOctetStringVarSizeAlias  BusOutputAsStruct=on
  o21 : Outport  Port=21  OutDataTypeStr=Bus: SeqOfSeqOfSeqOfVarSizeOctetStringVarSizeAlias  BusOutputAsStruct=on
  o22 : Outport  Port=22  OutDataTypeStr=Bus: SeqOfVarSizeEnumAlias  BusOutputAsStruct=on
  o23 : Outport  Port=23  OutDataTypeStr=Bus: SeqOfSeqOfVarSizeEnumAlias  BusOutputAsStruct=on
  o24 : Outport  Port=24  OutDataTypeStr=Bus: SeqOfSeqOfSeqOfVarSizeEnumAlias  BusOutputAsStruct=on
  o25 : Outport  Port=25  OutDataTypeStr=Bus: SeqOfVarSizeSeqAliases  BusOutputAsStruct=on
  o26 : Outport  Port=26  OutDataTypeStr=Bus: SeqOfSeqOfVarSizeSeqAliases  BusOutputAsStruct=on
  o27 : Outport  Port=27  OutDataTypeStr=Bus: SeqOfSeqOfSeqOfVarSizeSeqAliases  BusOutputAsStruct=on
  o28 : Outport  Port=28  OutDataTypeStr=Bus: SeqOfVarSizeSeqBuiltIn  BusOutputAsStruct=on
  o29 : Outport  Port=29  OutDataTypeStr=Bus: SeqOfSeqOfVarSizeSeqBuiltIn  BusOutputAsStruct=on
  o30 : Outport  Port=30  OutDataTypeStr=Bus: SeqOfSeqOfSeqOfVarSizeSeqBuiltIn  BusOutputAsStruct=on
  o31 : Outport  Port=31  OutDataTypeStr=Bus: SeqOfVarSizeChoiceAliases  BusOutputAsStruct=on
  o32 : Outport  Port=32  OutDataTypeStr=Bus: SeqOfSeqOfVarSizeChoiceAliases  BusOutputAsStruct=on
  o33 : Outport  Port=33  OutDataTypeStr=Bus: SeqOfSeqOfSeqOfVarSizeChoiceAliases  BusOutputAsStruct=on
  o34 : Outport  Port=34  OutDataTypeStr=Bus: SeqOfVarSizeChoiceBuiltIn  BusOutputAsStruct=on
  o35 : Outport  Port=35  OutDataTypeStr=Bus: SeqOfSeqOfVarSizeChoiceBuiltIn  BusOutputAsStruct=on
  o36 : Outport  Port=36  OutDataTypeStr=Bus: SeqOfSeqOfSeqOfVarSizeChoiceBuiltIn  BusOutputAsStruct=on
  wires:
  i1/1 -> i1_SeqOfVarSizeBoolAlias_BusSel/1
  i2/1 -> i2_SeqOfSeqOfVarSizeBoolAlias_BusSel/1
  i3/1 -> i3_SeqOfSeqOfSeqOfVarSizeBoolAlias_BusSel/1
  i4/1 -> i4_SeqOfVarSizeIntegerAlias_BusSel/1
  i5/1 -> i5_SeqOfSeqOfVarSizeIntegerAlias_BusSel/1
  i6/1 -> i6_SeqOfSeqOfSeqOfVarSizeIntegerAlias_BusSel/1
  i7/1 -> i7_SeqOfVarSizeRealAlias_BusSel/1
  i8/1 -> i8_SeqOfSeqOfVarSizeRealAlias_BusSel/1
  i9/1 -> i9_SeqOfSeqOfSeqOfVarSizeRealAlias_BusSel/1
  i10/1 -> i10_SeqOfVarSizeIA5StringFixedSizeAlias_BusSel/1
  i11/1 -> i11_SeqOfSeqOfVarSizeIA5StringFixedSizeAlias_BusSel/1
  i12/1 -> i12_SeqOfSeqOfSeqOfVarSizeIA5StringFixedSizeAlias_BusSel/1
  i13/1 -> i13_SeqOfVarSizeIA5StringVarSizeAlias_BusSel/1
  i14/1 -> i14_SeqOfSeqOfVarSizeIA5StringVarSizeAlias_BusSel/1
  i15/1 -> i15_SeqOfSeqOfSeqOfVarSizeIA5StringVarSizeAlias_BusSel/1
  i16/1 -> i16_SeqOfVarSizeOctetStringFixedSizeAlias_BusSel/1
  i17/1 -> i17_SeqOfSeqOfVarSizeOctetStringFixedSizeAlias_BusSel/1
  i18/1 -> i18_SeqOfSeqOfSeqOfVarSizeOctetStringFixedSizeAlias_BusSel/1
  i19/1 -> i19_SeqOfVarSizeOctetStringVarSizeAlias_BusSel/1
  i20/1 -> i20_SeqOfSeqOfVarSizeOctetStringVarSizeAlias_BusSel/1
  i21/1 -> i21_SeqOfSeqOfSeqOfVarSizeOctetStringVarSizeAlias_BusSel/1
  i22/1 -> i22_SeqOfVarSizeEnumAlias_BusSel/1
  i23/1 -> i23_SeqOfSeqOfVarSizeEnumAlias_BusSel/1
  i24/1 -> i24_SeqOfSeqOfSeqOfVarSizeEnumAlias_BusSel/1
  i25/1 -> i25_SeqOfVarSizeSeqAliases_BusSel/1
  i26/1 -> i26_SeqOfSeqOfVarSizeSeqAliases_BusSel/1
  i27/1 -> i27_SeqOfSeqOfSeqOfVarSizeSeqAliases_BusSel/1
  i28/1 -> i28_SeqOfVarSizeSeqBuiltIn_BusSel/1
  i29/1 -> i29_SeqOfSeqOfVarSizeSeqBuiltIn_BusSel/1
  i30/1 -> i30_SeqOfSeqOfSeqOfVarSizeSeqBuiltIn_BusSel/1
  i31/1 -> i31_SeqOfVarSizeChoiceAliases_BusSel/1
  i32/1 -> i32_SeqOfSeqOfVarSizeChoiceAliases_BusSel/1
  i33/1 -> i33_SeqOfSeqOfSeqOfVarSizeChoiceAliases_BusSel/1
  i34/1 -> i34_SeqOfVarSizeChoiceBuiltIn_BusSel/1
  i35/1 -> i35_SeqOfSeqOfVarSizeChoiceBuiltIn_BusSel/1
  i36/1 -> i36_SeqOfSeqOfSeqOfVarSizeChoiceBuiltIn_BusSel/1
  o1_SeqOfVarSizeBoolAlias_BusCre/1 -> o1/1
  o2_SeqOfSeqOfVarSizeBoolAlias_BusCre/1 -> o2/1
  o3_SeqOfSeqOfSeqOfVarSizeBoolAlias_BusCre/1 -> o3/1
  o4_SeqOfVarSizeIntegerAlias_BusCre/1 -> o4/1
  o5_SeqOfSeqOfVarSizeIntegerAlias_BusCre/1 -> o5/1
  o6_SeqOfSeqOfSeqOfVarSizeIntegerAlias_BusCre/1 -> o6/1
  o7_SeqOfVarSizeRealAlias_BusCre/1 -> o7/1
  o8_SeqOfSeqOfVarSizeRealAlias_BusCre/1 -> o8/1
  o9_SeqOfSeqOfSeqOfVarSizeRealAlias_BusCre/1 -> o9/1
  o10_SeqOfVarSizeIA5StringFixedSizeAlias_BusCre/1 -> o10/1
  o11_SeqOfSeqOfVarSizeIA5StringFixedSizeAlias_BusCre/1 -> o11/1
  o12_SeqOfSeqOfSeqOfVarSizeIA5StringFixedSizeAlias_BusCre/1 -> o12/1
  o13_SeqOfVarSizeIA5StringVarSizeAlias_BusCre/1 -> o13/1
  o14_SeqOfSeqOfVarSizeIA5StringVarSizeAlias_BusCre/1 -> o14/1
  o15_SeqOfSeqOfSeqOfVarSizeIA5StringVarSizeAlias_BusCre/1 -> o15/1
  o16_SeqOfVarSizeOctetStringFixedSizeAlias_BusCre/1 -> o16/1
  o17_SeqOfSeqOfVarSizeOctetStringFixedSizeAlias_BusCre/1 -> o17/1
  o18_SeqOfSeqOfSeqOfVarSizeOctetStringFixedSizeAlias_BusCre/1 -> o18/1
  o19_SeqOfVarSizeOctetStringVarSizeAlias_BusCre/1 -> o19/1
  o20_SeqOfSeqOfVarSizeOctetStringVarSizeAlias_BusCre/1 -> o20/1
  o21_SeqOfSeqOfSeqOfVarSizeOctetStringVarSizeAlias_BusCre/1 -> o21/1
  o22_SeqOfVarSizeEnumAlias_BusCre/1 -> o22/1
  o23_SeqOfSeqOfVarSizeEnumAlias_BusCre/1 -> o23/1
  o24_SeqOfSeqOfSeqOfVarSizeEnumAlias_BusCre/1 -> o24/1
  o25_SeqOfVarSizeSeqAliases_BusCre/1 -> o25/1
  o26_SeqOfSeqOfVarSizeSeqAliases_BusCre/1 -> o26/1
  o27_SeqOfSeqOfSeqOfVarSizeSeqAliases_BusCre/1 -> o27/1
  o28_SeqOfVarSizeSeqBuiltIn_BusCre/1 -> o28/1
  o29_SeqOfSeqOfVarSizeSeqBuiltIn_BusCre/1 -> o29/1
  o30_SeqOfSeqOfSeqOfVarSizeSeqBuiltIn_BusCre/1 -> o30/1
  o31_SeqOfVarSizeChoiceAliases_BusCre/1 -> o31/1
  o32_SeqOfSeqOfVarSizeChoiceAliases_BusCre/1 -> o32/1
  o33_SeqOfSeqOfSeqOfVarSizeChoiceAliases_BusCre/1 -> o33/1
  o34_SeqOfVarSizeChoiceBuiltIn_BusCre/1 -> o34/1
  o35_SeqOfSeqOfVarSizeChoiceBuiltIn_BusCre/1 -> o35/1
  o36_SeqOfSeqOfSeqOfVarSizeChoiceBuiltIn_BusCre/1 -> o36/1
  i36_SeqOfSeqOfSeqOfVarSizeChoiceBuiltIn_BusSel/1 -> o36_SeqOfSeqOfSeqOfVarSizeChoiceBuiltIn_BusCre/1  "<arr>"
  i36_SeqOfSeqOfSeqOfVarSizeChoiceBuiltIn_BusSel/2 -> o36_SeqOfSeqOfSeqOfVarSizeChoiceBuiltIn_BusCre/2  "<nCount>"
  i35_SeqOfSeqOfVarSizeChoiceBuiltIn_BusSel/1 -> o35_SeqOfSeqOfVarSizeChoiceBuiltIn_BusCre/1  "<arr>"
  i35_SeqOfSeqOfVarSizeChoiceBuiltIn_BusSel/2 -> o35_SeqOfSeqOfVarSizeChoiceBuiltIn_BusCre/2  "<nCount>"
  i34_SeqOfVarSizeChoiceBuiltIn_BusSel/1 -> o34_SeqOfVarSizeChoiceBuiltIn_BusCre/1  "<arr>"
  i34_SeqOfVarSizeChoiceBuiltIn_BusSel/2 -> o34_SeqOfVarSizeChoiceBuiltIn_BusCre/2  "<nCount>"
  i33_SeqOfSeqOfSeqOfVarSizeChoiceAliases_BusSel/1 -> o33_SeqOfSeqOfSeqOfVarSizeChoiceAliases_BusCre/1  "<arr>"
  i33_SeqOfSeqOfSeqOfVarSizeChoiceAliases_BusSel/2 -> o33_SeqOfSeqOfSeqOfVarSizeChoiceAliases_BusCre/2  "<nCount>"
  i32_SeqOfSeqOfVarSizeChoiceAliases_BusSel/1 -> o32_SeqOfSeqOfVarSizeChoiceAliases_BusCre/1  "<arr>"
  i32_SeqOfSeqOfVarSizeChoiceAliases_BusSel/2 -> o32_SeqOfSeqOfVarSizeChoiceAliases_BusCre/2  "<nCount>"
  i31_SeqOfVarSizeChoiceAliases_BusSel/1 -> o31_SeqOfVarSizeChoiceAliases_BusCre/1  "<arr>"
  i31_SeqOfVarSizeChoiceAliases_BusSel/2 -> o31_SeqOfVarSizeChoiceAliases_BusCre/2  "<nCount>"
  o23_SeqOfSeqOfVarSizeEnumAlias_BusCre1/1 -> QgencimplseqofvariablesizeRi_Seqofvariablesizeiface/23
  o4_SeqOfVarSizeIntegerAlias_BusCre1/1 -> QgencimplseqofvariablesizeRi_Seqofvariablesizeiface/4
  o29_SeqOfSeqOfVarSizeSeqBuiltIn_BusCre1/1 -> QgencimplseqofvariablesizeRi_Seqofvariablesizeiface/29
  o8_SeqOfSeqOfVarSizeRealAlias_BusCre1/1 -> QgencimplseqofvariablesizeRi_Seqofvariablesizeiface/8
  o17_SeqOfSeqOfVarSizeOctetStringFixedSizeAlias_BusCre1/1 -> QgencimplseqofvariablesizeRi_Seqofvariablesizeiface/17
  o26_SeqOfSeqOfVarSizeSeqAliases_BusCre1/1 -> QgencimplseqofvariablesizeRi_Seqofvariablesizeiface/26
  o24_SeqOfSeqOfSeqOfVarSizeEnumAlias_BusCre1/1 -> QgencimplseqofvariablesizeRi_Seqofvariablesizeiface/24
  o27_SeqOfSeqOfSeqOfVarSizeSeqAliases_BusCre1/1 -> QgencimplseqofvariablesizeRi_Seqofvariablesizeiface/27
  o15_SeqOfSeqOfSeqOfVarSizeIA5StringVarSizeAlias_BusCre1/1 -> QgencimplseqofvariablesizeRi_Seqofvariablesizeiface/15
  o21_SeqOfSeqOfSeqOfVarSizeOctetStringVarSizeAlias_BusCre1/1 -> QgencimplseqofvariablesizeRi_Seqofvariablesizeiface/21
  o18_SeqOfSeqOfSeqOfVarSizeOctetStringFixedSizeAlias_BusCre1/1 -> QgencimplseqofvariablesizeRi_Seqofvariablesizeiface/18
  o30_SeqOfSeqOfSeqOfVarSizeSeqBuiltIn_BusCre1/1 -> QgencimplseqofvariablesizeRi_Seqofvariablesizeiface/30
  o13_SeqOfVarSizeIA5StringVarSizeAlias_BusCre1/1 -> QgencimplseqofvariablesizeRi_Seqofvariablesizeiface/13
  o28_SeqOfVarSizeSeqBuiltIn_BusCre1/1 -> QgencimplseqofvariablesizeRi_Seqofvariablesizeiface/28
  o20_SeqOfSeqOfVarSizeOctetStringVarSizeAlias_BusCre1/1 -> QgencimplseqofvariablesizeRi_Seqofvariablesizeiface/20
  o19_SeqOfVarSizeOctetStringVarSizeAlias_BusCre1/1 -> QgencimplseqofvariablesizeRi_Seqofvariablesizeiface/19
  o5_SeqOfSeqOfVarSizeIntegerAlias_BusCre1/1 -> QgencimplseqofvariablesizeRi_Seqofvariablesizeiface/5
  o10_SeqOfVarSizeIA5StringFixedSizeAlias_BusCre1/1 -> QgencimplseqofvariablesizeRi_Seqofvariablesizeiface/10
  o22_SeqOfVarSizeEnumAlias_BusCre1/1 -> QgencimplseqofvariablesizeRi_Seqofvariablesizeiface/22
  o12_SeqOfSeqOfSeqOfVarSizeIA5StringFixedSizeAlias_BusCre1/1 -> QgencimplseqofvariablesizeRi_Seqofvariablesizeiface/12
  o9_SeqOfSeqOfSeqOfVarSizeRealAlias_BusCre1/1 -> QgencimplseqofvariablesizeRi_Seqofvariablesizeiface/9
  o6_SeqOfSeqOfSeqOfVarSizeIntegerAlias_BusCre1/1 -> QgencimplseqofvariablesizeRi_Seqofvariablesizeiface/6
  o11_SeqOfSeqOfVarSizeIA5StringFixedSizeAlias_BusCre1/1 -> QgencimplseqofvariablesizeRi_Seqofvariablesizeiface/11
  o7_SeqOfVarSizeRealAlias_BusCre1/1 -> QgencimplseqofvariablesizeRi_Seqofvariablesizeiface/7
  o1_SeqOfVarSizeBoolAlias_BusCre1/1 -> QgencimplseqofvariablesizeRi_Seqofvariablesizeiface/1
  o16_SeqOfVarSizeOctetStringFixedSizeAlias_BusCre1/1 -> QgencimplseqofvariablesizeRi_Seqofvariablesizeiface/16
  o14_SeqOfSeqOfVarSizeIA5StringVarSizeAlias_BusCre1/1 -> QgencimplseqofvariablesizeRi_Seqofvariablesizeiface/14
  o2_SeqOfSeqOfVarSizeBoolAlias_BusCre1/1 -> QgencimplseqofvariablesizeRi_Seqofvariablesizeiface/2
  o3_SeqOfSeqOfSeqOfVarSizeBoolAlias_BusCre1/1 -> QgencimplseqofvariablesizeRi_Seqofvariablesizeiface/3
  o25_SeqOfVarSizeSeqAliases_BusCre1/1 -> QgencimplseqofvariablesizeRi_Seqofvariablesizeiface/25
  i1_SeqOfVarSizeBoolAlias_BusSel/1 -> o1_SeqOfVarSizeBoolAlias_BusCre1/1  "<arr>"
  i1_SeqOfVarSizeBoolAlias_BusSel/2 -> o1_SeqOfVarSizeBoolAlias_BusCre1/2  "<nCount>"
  i2_SeqOfSeqOfVarSizeBoolAlias_BusSel/1 -> o2_SeqOfSeqOfVarSizeBoolAlias_BusCre1/1  "<arr>"
  i2_SeqOfSeqOfVarSizeBoolAlias_BusSel/2 -> o2_SeqOfSeqOfVarSizeBoolAlias_BusCre1/2  "<nCount>"
  i3_SeqOfSeqOfSeqOfVarSizeBoolAlias_BusSel/1 -> o3_SeqOfSeqOfSeqOfVarSizeBoolAlias_BusCre1/1  "<arr>"
  i3_SeqOfSeqOfSeqOfVarSizeBoolAlias_BusSel/2 -> o3_SeqOfSeqOfSeqOfVarSizeBoolAlias_BusCre1/2  "<nCount>"
  i4_SeqOfVarSizeIntegerAlias_BusSel/1 -> o4_SeqOfVarSizeIntegerAlias_BusCre1/1  "<arr>"
  i4_SeqOfVarSizeIntegerAlias_BusSel/2 -> o4_SeqOfVarSizeIntegerAlias_BusCre1/2  "<nCount>"
  i5_SeqOfSeqOfVarSizeIntegerAlias_BusSel/1 -> o5_SeqOfSeqOfVarSizeIntegerAlias_BusCre1/1  "<arr>"
  i5_SeqOfSeqOfVarSizeIntegerAlias_BusSel/2 -> o5_SeqOfSeqOfVarSizeIntegerAlias_BusCre1/2  "<nCount>"
  i6_SeqOfSeqOfSeqOfVarSizeIntegerAlias_BusSel/1 -> o6_SeqOfSeqOfSeqOfVarSizeIntegerAlias_BusCre1/1  "<arr>"
  i6_SeqOfSeqOfSeqOfVarSizeIntegerAlias_BusSel/2 -> o6_SeqOfSeqOfSeqOfVarSizeIntegerAlias_BusCre1/2  "<nCount>"
  i7_SeqOfVarSizeRealAlias_BusSel/1 -> o7_SeqOfVarSizeRealAlias_BusCre1/1  "<arr>"
  i7_SeqOfVarSizeRealAlias_BusSel/2 -> o7_SeqOfVarSizeRealAlias_BusCre1/2  "<nCount>"
  i8_SeqOfSeqOfVarSizeRealAlias_BusSel/1 -> o8_SeqOfSeqOfVarSizeRealAlias_BusCre1/1  "<arr>"
  i8_SeqOfSeqOfVarSizeRealAlias_BusSel/2 -> o8_SeqOfSeqOfVarSizeRealAlias_BusCre1/2  "<nCount>"
  i9_SeqOfSeqOfSeqOfVarSizeRealAlias_BusSel/1 -> o9_SeqOfSeqOfSeqOfVarSizeRealAlias_BusCre1/1  "<arr>"
  i9_SeqOfSeqOfSeqOfVarSizeRealAlias_BusSel/2 -> o9_SeqOfSeqOfSeqOfVarSizeRealAlias_BusCre1/2  "<nCount>"
  i10_SeqOfVarSizeIA5StringFixedSizeAlias_BusSel/1 -> o10_SeqOfVarSizeIA5StringFixedSizeAlias_BusCre1/1  "<arr>"
  i10_SeqOfVarSizeIA5StringFixedSizeAlias_BusSel/2 -> o10_SeqOfVarSizeIA5StringFixedSizeAlias_BusCre1/2  "<nCount>"
  i11_SeqOfSeqOfVarSizeIA5StringFixedSizeAlias_BusSel/1 -> o11_SeqOfSeqOfVarSizeIA5StringFixedSizeAlias_BusCre1/1  "<arr>"
  i11_SeqOfSeqOfVarSizeIA5StringFixedSizeAlias_BusSel/2 -> o11_SeqOfSeqOfVarSizeIA5StringFixedSizeAlias_BusCre1/2  "<nCount>"
  i12_SeqOfSeqOfSeqOfVarSizeIA5StringFixedSizeAlias_BusSel/1 -> o12_SeqOfSeqOfSeqOfVarSizeIA5StringFixedSizeAlias_BusCre1/1  "<arr>"
  i12_SeqOfSeqOfSeqOfVarSizeIA5StringFixedSizeAlias_BusSel/2 -> o12_SeqOfSeqOfSeqOfVarSizeIA5StringFixedSizeAlias_BusCre1/2  "<nCount>"
  i13_SeqOfVarSizeIA5StringVarSizeAlias_BusSel/1 -> o13_SeqOfVarSizeIA5StringVarSizeAlias_BusCre1/1  "<arr>"
  i13_SeqOfVarSizeIA5StringVarSizeAlias_BusSel/2 -> o13_SeqOfVarSizeIA5StringVarSizeAlias_BusCre1/2  "<nCount>"
  i14_SeqOfSeqOfVarSizeIA5StringVarSizeAlias_BusSel/1 -> o14_SeqOfSeqOfVarSizeIA5StringVarSizeAlias_BusCre1/1  "<arr>"
  i14_SeqOfSeqOfVarSizeIA5StringVarSizeAlias_BusSel/2 -> o14_SeqOfSeqOfVarSizeIA5StringVarSizeAlias_BusCre1/2  "<nCount>"
  i15_SeqOfSeqOfSeqOfVarSizeIA5StringVarSizeAlias_BusSel/1 -> o15_SeqOfSeqOfSeqOfVarSizeIA5StringVarSizeAlias_BusCre1/1  "<arr>"
  i15_SeqOfSeqOfSeqOfVarSizeIA5StringVarSizeAlias_BusSel/2 -> o15_SeqOfSeqOfSeqOfVarSizeIA5StringVarSizeAlias_BusCre1/2  "<nCount>"
  i16_SeqOfVarSizeOctetStringFixedSizeAlias_BusSel/1 -> o16_SeqOfVarSizeOctetStringFixedSizeAlias_BusCre1/1  "<arr>"
  i16_SeqOfVarSizeOctetStringFixedSizeAlias_BusSel/2 -> o16_SeqOfVarSizeOctetStringFixedSizeAlias_BusCre1/2  "<nCount>"
  i17_SeqOfSeqOfVarSizeOctetStringFixedSizeAlias_BusSel/1 -> o17_SeqOfSeqOfVarSizeOctetStringFixedSizeAlias_BusCre1/1  "<arr>"
  i17_SeqOfSeqOfVarSizeOctetStringFixedSizeAlias_BusSel/2 -> o17_SeqOfSeqOfVarSizeOctetStringFixedSizeAlias_BusCre1/2  "<nCount>"
  i18_SeqOfSeqOfSeqOfVarSizeOctetStringFixedSizeAlias_BusSel/1 -> o18_SeqOfSeqOfSeqOfVarSizeOctetStringFixedSizeAlias_BusCre1/1  "<arr>"
  i18_SeqOfSeqOfSeqOfVarSizeOctetStringFixedSizeAlias_BusSel/2 -> o18_SeqOfSeqOfSeqOfVarSizeOctetStringFixedSizeAlias_BusCre1/2  "<nCount>"
  i19_SeqOfVarSizeOctetStringVarSizeAlias_BusSel/1 -> o19_SeqOfVarSizeOctetStringVarSizeAlias_BusCre1/1  "<arr>"
  i19_SeqOfVarSizeOctetStringVarSizeAlias_BusSel/2 -> o19_SeqOfVarSizeOctetStringVarSizeAlias_BusCre1/2  "<nCount>"
  i20_SeqOfSeqOfVarSizeOctetStringVarSizeAlias_BusSel/1 -> o20_SeqOfSeqOfVarSizeOctetStringVarSizeAlias_BusCre1/1  "<arr>"
  i20_SeqOfSeqOfVarSizeOctetStringVarSizeAlias_BusSel/2 -> o20_SeqOfSeqOfVarSizeOctetStringVarSizeAlias_BusCre1/2  "<nCount>"
  i21_SeqOfSeqOfSeqOfVarSizeOctetStringVarSizeAlias_BusSel/1 -> o21_SeqOfSeqOfSeqOfVarSizeOctetStringVarSizeAlias_BusCre1/1  "<arr>"
  i21_SeqOfSeqOfSeqOfVarSizeOctetStringVarSizeAlias_BusSel/2 -> o21_SeqOfSeqOfSeqOfVarSizeOctetStringVarSizeAlias_BusCre1/2  "<nCount>"
  i22_SeqOfVarSizeEnumAlias_BusSel/1 -> o22_SeqOfVarSizeEnumAlias_BusCre1/1  "<arr>"
  i22_SeqOfVarSizeEnumAlias_BusSel/2 -> o22_SeqOfVarSizeEnumAlias_BusCre1/2  "<nCount>"
  i23_SeqOfSeqOfVarSizeEnumAlias_BusSel/1 -> o23_SeqOfSeqOfVarSizeEnumAlias_BusCre1/1  "<arr>"
  i23_SeqOfSeqOfVarSizeEnumAlias_BusSel/2 -> o23_SeqOfSeqOfVarSizeEnumAlias_BusCre1/2  "<nCount>"
  i24_SeqOfSeqOfSeqOfVarSizeEnumAlias_BusSel/1 -> o24_SeqOfSeqOfSeqOfVarSizeEnumAlias_BusCre1/1  "<arr>"
  i24_SeqOfSeqOfSeqOfVarSizeEnumAlias_BusSel/2 -> o24_SeqOfSeqOfSeqOfVarSizeEnumAlias_BusCre1/2  "<nCount>"
  i25_SeqOfVarSizeSeqAliases_BusSel/1 -> o25_SeqOfVarSizeSeqAliases_BusCre1/1  "<arr>"
  i25_SeqOfVarSizeSeqAliases_BusSel/2 -> o25_SeqOfVarSizeSeqAliases_BusCre1/2  "<nCount>"
  i26_SeqOfSeqOfVarSizeSeqAliases_BusSel/1 -> o26_SeqOfSeqOfVarSizeSeqAliases_BusCre1/1  "<arr>"
  i26_SeqOfSeqOfVarSizeSeqAliases_BusSel/2 -> o26_SeqOfSeqOfVarSizeSeqAliases_BusCre1/2  "<nCount>"
  i27_SeqOfSeqOfSeqOfVarSizeSeqAliases_BusSel/1 -> o27_SeqOfSeqOfSeqOfVarSizeSeqAliases_BusCre1/1  "<arr>"
  i27_SeqOfSeqOfSeqOfVarSizeSeqAliases_BusSel/2 -> o27_SeqOfSeqOfSeqOfVarSizeSeqAliases_BusCre1/2  "<nCount>"
  i28_SeqOfVarSizeSeqBuiltIn_BusSel/1 -> o28_SeqOfVarSizeSeqBuiltIn_BusCre1/1  "<arr>"
  i28_SeqOfVarSizeSeqBuiltIn_BusSel/2 -> o28_SeqOfVarSizeSeqBuiltIn_BusCre1/2  "<nCount>"
  i29_SeqOfSeqOfVarSizeSeqBuiltIn_BusSel/1 -> o29_SeqOfSeqOfVarSizeSeqBuiltIn_BusCre1/1  "<arr>"
  i29_SeqOfSeqOfVarSizeSeqBuiltIn_BusSel/2 -> o29_SeqOfSeqOfVarSizeSeqBuiltIn_BusCre1/2  "<nCount>"
  i30_SeqOfSeqOfSeqOfVarSizeSeqBuiltIn_BusSel/1 -> o30_SeqOfSeqOfSeqOfVarSizeSeqBuiltIn_BusCre1/1  "<arr>"
  i30_SeqOfSeqOfSeqOfVarSizeSeqBuiltIn_BusSel/2 -> o30_SeqOfSeqOfSeqOfVarSizeSeqBuiltIn_BusCre1/2  "<nCount>"
  i8_SeqOfSeqOfVarSizeRealAlias_BusSel1/1 -> o8_SeqOfSeqOfVarSizeRealAlias_BusCre/1  "<arr>"
  i8_SeqOfSeqOfVarSizeRealAlias_BusSel1/2 -> o8_SeqOfSeqOfVarSizeRealAlias_BusCre/2  "<nCount>"
  i6_SeqOfSeqOfSeqOfVarSizeIntegerAlias_BusSel1/2 -> o6_SeqOfSeqOfSeqOfVarSizeIntegerAlias_BusCre/2  "<nCount>"
  i6_SeqOfSeqOfSeqOfVarSizeIntegerAlias_BusSel1/1 -> o6_SeqOfSeqOfSeqOfVarSizeIntegerAlias_BusCre/1  "<arr>"
  i7_SeqOfVarSizeRealAlias_BusSel1/2 -> o7_SeqOfVarSizeRealAlias_BusCre/2  "<nCount>"
  i7_SeqOfVarSizeRealAlias_BusSel1/1 -> o7_SeqOfVarSizeRealAlias_BusCre/1  "<arr>"
  i9_SeqOfSeqOfSeqOfVarSizeRealAlias_BusSel1/1 -> o9_SeqOfSeqOfSeqOfVarSizeRealAlias_BusCre/1  "<arr>"
  i9_SeqOfSeqOfSeqOfVarSizeRealAlias_BusSel1/2 -> o9_SeqOfSeqOfSeqOfVarSizeRealAlias_BusCre/2  "<nCount>"
  QgencimplseqofvariablesizeRi_Seqofvariablesizeiface/17 -> i17_SeqOfSeqOfVarSizeOctetStringFixedSizeAlias_BusSel1/1
  QgencimplseqofvariablesizeRi_Seqofvariablesizeiface/27 -> i27_SeqOfSeqOfSeqOfVarSizeSeqAliases_BusSel1/1
  QgencimplseqofvariablesizeRi_Seqofvariablesizeiface/9 -> i9_SeqOfSeqOfSeqOfVarSizeRealAlias_BusSel1/1
  QgencimplseqofvariablesizeRi_Seqofvariablesizeiface/10 -> i10_SeqOfVarSizeIA5StringFixedSizeAlias_BusSel1/1
  QgencimplseqofvariablesizeRi_Seqofvariablesizeiface/30 -> i30_SeqOfSeqOfSeqOfVarSizeSeqBuiltIn_BusSel1/1
  QgencimplseqofvariablesizeRi_Seqofvariablesizeiface/28 -> i28_SeqOfVarSizeSeqBuiltIn_BusSel1/1
  QgencimplseqofvariablesizeRi_Seqofvariablesizeiface/26 -> i26_SeqOfSeqOfVarSizeSeqAliases_BusSel1/1
  QgencimplseqofvariablesizeRi_Seqofvariablesizeiface/21 -> i21_SeqOfSeqOfSeqOfVarSizeOctetStringVarSizeAlias_BusSel1/1
  QgencimplseqofvariablesizeRi_Seqofvariablesizeiface/23 -> i23_SeqOfSeqOfVarSizeEnumAlias_BusSel1/1
  QgencimplseqofvariablesizeRi_Seqofvariablesizeiface/25 -> i25_SeqOfVarSizeSeqAliases_BusSel1/1
  QgencimplseqofvariablesizeRi_Seqofvariablesizeiface/20 -> i20_SeqOfSeqOfVarSizeOctetStringVarSizeAlias_BusSel1/1
  QgencimplseqofvariablesizeRi_Seqofvariablesizeiface/13 -> i13_SeqOfVarSizeIA5StringVarSizeAlias_BusSel1/1
  QgencimplseqofvariablesizeRi_Seqofvariablesizeiface/19 -> i19_SeqOfVarSizeOctetStringVarSizeAlias_BusSel1/1
  QgencimplseqofvariablesizeRi_Seqofvariablesizeiface/18 -> i18_SeqOfSeqOfSeqOfVarSizeOctetStringFixedSizeAlias_BusSel1/1
  QgencimplseqofvariablesizeRi_Seqofvariablesizeiface/5 -> i5_SeqOfSeqOfVarSizeIntegerAlias_BusSel1/1
  QgencimplseqofvariablesizeRi_Seqofvariablesizeiface/8 -> i8_SeqOfSeqOfVarSizeRealAlias_BusSel1/1
  QgencimplseqofvariablesizeRi_Seqofvariablesizeiface/6 -> i6_SeqOfSeqOfSeqOfVarSizeIntegerAlias_BusSel1/1
  QgencimplseqofvariablesizeRi_Seqofvariablesizeiface/2 -> i2_SeqOfSeqOfVarSizeBoolAlias_BusSel1/1
  QgencimplseqofvariablesizeRi_Seqofvariablesizeiface/7 -> i7_SeqOfVarSizeRealAlias_BusSel1/1
  QgencimplseqofvariablesizeRi_Seqofvariablesizeiface/1 -> i1_SeqOfVarSizeBoolAlias_BusSel1/1
  QgencimplseqofvariablesizeRi_Seqofvariablesizeiface/12 -> i12_SeqOfSeqOfSeqOfVarSizeIA5StringFixedSizeAlias_BusSel1/1
  QgencimplseqofvariablesizeRi_Seqofvariablesizeiface/15 -> i15_SeqOfSeqOfSeqOfVarSizeIA5StringVarSizeAlias_BusSel1/1
  QgencimplseqofvariablesizeRi_Seqofvariablesizeiface/29 -> i29_SeqOfSeqOfVarSizeSeqBuiltIn_BusSel1/1
  i22_SeqOfVarSizeEnumAlias_BusSel1/2 -> o22_SeqOfVarSizeEnumAlias_BusCre/2  "<nCount>"
  QgencimplseqofvariablesizeRi_Seqofvariablesizeiface/3 -> i3_SeqOfSeqOfSeqOfVarSizeBoolAlias_BusSel1/1
  i30_SeqOfSeqOfSeqOfVarSizeSeqBuiltIn_BusSel1/2 -> o30_SeqOfSeqOfSeqOfVarSizeSeqBuiltIn_BusCre/2  "<nCount>"
  i29_SeqOfSeqOfVarSizeSeqBuiltIn_BusSel1/2 -> o29_SeqOfSeqOfVarSizeSeqBuiltIn_BusCre/2  "<nCount>"
  i29_SeqOfSeqOfVarSizeSeqBuiltIn_BusSel1/1 -> o29_SeqOfSeqOfVarSizeSeqBuiltIn_BusCre/1  "<arr>"
  i28_SeqOfVarSizeSeqBuiltIn_BusSel1/2 -> o28_SeqOfVarSizeSeqBuiltIn_BusCre/2  "<nCount>"
  i27_SeqOfSeqOfSeqOfVarSizeSeqAliases_BusSel1/1 -> o27_SeqOfSeqOfSeqOfVarSizeSeqAliases_BusCre/1  "<arr>"
  i30_SeqOfSeqOfSeqOfVarSizeSeqBuiltIn_BusSel1/1 -> o30_SeqOfSeqOfSeqOfVarSizeSeqBuiltIn_BusCre/1  "<arr>"
  i28_SeqOfVarSizeSeqBuiltIn_BusSel1/1 -> o28_SeqOfVarSizeSeqBuiltIn_BusCre/1  "<arr>"
  i25_SeqOfVarSizeSeqAliases_BusSel1/2 -> o25_SeqOfVarSizeSeqAliases_BusCre/2  "<nCount>"
  i24_SeqOfSeqOfSeqOfVarSizeEnumAlias_BusSel1/2 -> o24_SeqOfSeqOfSeqOfVarSizeEnumAlias_BusCre/2  "<nCount>"
  QgencimplseqofvariablesizeRi_Seqofvariablesizeiface/24 -> i24_SeqOfSeqOfSeqOfVarSizeEnumAlias_BusSel1/1
  i23_SeqOfSeqOfVarSizeEnumAlias_BusSel1/2 -> o23_SeqOfSeqOfVarSizeEnumAlias_BusCre/2  "<nCount>"
  i20_SeqOfSeqOfVarSizeOctetStringVarSizeAlias_BusSel1/2 -> o20_SeqOfSeqOfVarSizeOctetStringVarSizeAlias_BusCre/2  "<nCount>"
  i23_SeqOfSeqOfVarSizeEnumAlias_BusSel1/1 -> o23_SeqOfSeqOfVarSizeEnumAlias_BusCre/1  "<arr>"
  i20_SeqOfSeqOfVarSizeOctetStringVarSizeAlias_BusSel1/1 -> o20_SeqOfSeqOfVarSizeOctetStringVarSizeAlias_BusCre/1  "<arr>"
  i19_SeqOfVarSizeOctetStringVarSizeAlias_BusSel1/2 -> o19_SeqOfVarSizeOctetStringVarSizeAlias_BusCre/2  "<nCount>"
  i14_SeqOfSeqOfVarSizeIA5StringVarSizeAlias_BusSel1/1 -> o14_SeqOfSeqOfVarSizeIA5StringVarSizeAlias_BusCre/1  "<arr>"
  i17_SeqOfSeqOfVarSizeOctetStringFixedSizeAlias_BusSel1/2 -> o17_SeqOfSeqOfVarSizeOctetStringFixedSizeAlias_BusCre/2  "<nCount>"
  i26_SeqOfSeqOfVarSizeSeqAliases_BusSel1/1 -> o26_SeqOfSeqOfVarSizeSeqAliases_BusCre/1  "<arr>"
  QgencimplseqofvariablesizeRi_Seqofvariablesizeiface/14 -> i14_SeqOfSeqOfVarSizeIA5StringVarSizeAlias_BusSel1/1
  i13_SeqOfVarSizeIA5StringVarSizeAlias_BusSel1/1 -> o13_SeqOfVarSizeIA5StringVarSizeAlias_BusCre/1  "<arr>"
  QgencimplseqofvariablesizeRi_Seqofvariablesizeiface/11 -> i11_SeqOfSeqOfVarSizeIA5StringFixedSizeAlias_BusSel1/1
  i18_SeqOfSeqOfSeqOfVarSizeOctetStringFixedSizeAlias_BusSel1/1 -> o18_SeqOfSeqOfSeqOfVarSizeOctetStringFixedSizeAlias_BusCre/1  "<arr>"
  i18_SeqOfSeqOfSeqOfVarSizeOctetStringFixedSizeAlias_BusSel1/2 -> o18_SeqOfSeqOfSeqOfVarSizeOctetStringFixedSizeAlias_BusCre/2  "<nCount>"
  i17_SeqOfSeqOfVarSizeOctetStringFixedSizeAlias_BusSel1/1 -> o17_SeqOfSeqOfVarSizeOctetStringFixedSizeAlias_BusCre/1  "<arr>"
  i15_SeqOfSeqOfSeqOfVarSizeIA5StringVarSizeAlias_BusSel1/1 -> o15_SeqOfSeqOfSeqOfVarSizeIA5StringVarSizeAlias_BusCre/1  "<arr>"
  i4_SeqOfVarSizeIntegerAlias_BusSel1/2 -> o4_SeqOfVarSizeIntegerAlias_BusCre/2  "<nCount>"
  i21_SeqOfSeqOfSeqOfVarSizeOctetStringVarSizeAlias_BusSel1/1 -> o21_SeqOfSeqOfSeqOfVarSizeOctetStringVarSizeAlias_BusCre/1  "<arr>"
  QgencimplseqofvariablesizeRi_Seqofvariablesizeiface/16 -> i16_SeqOfVarSizeOctetStringFixedSizeAlias_BusSel1/1
  i4_SeqOfVarSizeIntegerAlias_BusSel1/1 -> o4_SeqOfVarSizeIntegerAlias_BusCre/1  "<arr>"
  i19_SeqOfVarSizeOctetStringVarSizeAlias_BusSel1/1 -> o19_SeqOfVarSizeOctetStringVarSizeAlias_BusCre/1  "<arr>"
  i5_SeqOfSeqOfVarSizeIntegerAlias_BusSel1/2 -> o5_SeqOfSeqOfVarSizeIntegerAlias_BusCre/2  "<nCount>"
  i5_SeqOfSeqOfVarSizeIntegerAlias_BusSel1/1 -> o5_SeqOfSeqOfVarSizeIntegerAlias_BusCre/1  "<arr>"
  i3_SeqOfSeqOfSeqOfVarSizeBoolAlias_BusSel1/2 -> o3_SeqOfSeqOfSeqOfVarSizeBoolAlias_BusCre/2  "<nCount>"
  i12_SeqOfSeqOfSeqOfVarSizeIA5StringFixedSizeAlias_BusSel1/2 -> o12_SeqOfSeqOfSeqOfVarSizeIA5StringFixedSizeAlias_BusCre/2  "<nCount>"
  QgencimplseqofvariablesizeRi_Seqofvariablesizeiface/4 -> i4_SeqOfVarSizeIntegerAlias_BusSel1/1
  i11_SeqOfSeqOfVarSizeIA5StringFixedSizeAlias_BusSel1/1 -> o11_SeqOfSeqOfVarSizeIA5StringFixedSizeAlias_BusCre/1  "<arr>"
  i11_SeqOfSeqOfVarSizeIA5StringFixedSizeAlias_BusSel1/2 -> o11_SeqOfSeqOfVarSizeIA5StringFixedSizeAlias_BusCre/2  "<nCount>"
  i12_SeqOfSeqOfSeqOfVarSizeIA5StringFixedSizeAlias_BusSel1/1 -> o12_SeqOfSeqOfSeqOfVarSizeIA5StringFixedSizeAlias_BusCre/1  "<arr>"
  i2_SeqOfSeqOfVarSizeBoolAlias_BusSel1/2 -> o2_SeqOfSeqOfVarSizeBoolAlias_BusCre/2  "<nCount>"
  i26_SeqOfSeqOfVarSizeSeqAliases_BusSel1/2 -> o26_SeqOfSeqOfVarSizeSeqAliases_BusCre/2  "<nCount>"
  i27_SeqOfSeqOfSeqOfVarSizeSeqAliases_BusSel1/2 -> o27_SeqOfSeqOfSeqOfVarSizeSeqAliases_BusCre/2  "<nCount>"
  i21_SeqOfSeqOfSeqOfVarSizeOctetStringVarSizeAlias_BusSel1/2 -> o21_SeqOfSeqOfSeqOfVarSizeOctetStringVarSizeAlias_BusCre/2  "<nCount>"
  i15_SeqOfSeqOfSeqOfVarSizeIA5StringVarSizeAlias_BusSel1/2 -> o15_SeqOfSeqOfSeqOfVarSizeIA5StringVarSizeAlias_BusCre/2  "<nCount>"
  i2_SeqOfSeqOfVarSizeBoolAlias_BusSel1/1 -> o2_SeqOfSeqOfVarSizeBoolAlias_BusCre/1  "<arr>"
  i16_SeqOfVarSizeOctetStringFixedSizeAlias_BusSel1/2 -> o16_SeqOfVarSizeOctetStringFixedSizeAlias_BusCre/2  "<nCount>"
  QgencimplseqofvariablesizeRi_Seqofvariablesizeiface/22 -> i22_SeqOfVarSizeEnumAlias_BusSel1/1
  i3_SeqOfSeqOfSeqOfVarSizeBoolAlias_BusSel1/1 -> o3_SeqOfSeqOfSeqOfVarSizeBoolAlias_BusCre/1  "<arr>"
  i24_SeqOfSeqOfSeqOfVarSizeEnumAlias_BusSel1/1 -> o24_SeqOfSeqOfSeqOfVarSizeEnumAlias_BusCre/1  "<arr>"
  i14_SeqOfSeqOfVarSizeIA5StringVarSizeAlias_BusSel1/2 -> o14_SeqOfSeqOfVarSizeIA5StringVarSizeAlias_BusCre/2  "<nCount>"
  i1_SeqOfVarSizeBoolAlias_BusSel1/1 -> o1_SeqOfVarSizeBoolAlias_BusCre/1  "<arr>"
  i25_SeqOfVarSizeSeqAliases_BusSel1/1 -> o25_SeqOfVarSizeSeqAliases_BusCre/1  "<arr>"
  i1_SeqOfVarSizeBoolAlias_BusSel1/2 -> o1_SeqOfVarSizeBoolAlias_BusCre/2  "<nCount>"
  i10_SeqOfVarSizeIA5StringFixedSizeAlias_BusSel1/2 -> o10_SeqOfVarSizeIA5StringFixedSizeAlias_BusCre/2  "<nCount>"
  i13_SeqOfVarSizeIA5StringVarSizeAlias_BusSel1/2 -> o13_SeqOfVarSizeIA5StringVarSizeAlias_BusCre/2  "<nCount>"
  i10_SeqOfVarSizeIA5StringFixedSizeAlias_BusSel1/1 -> o10_SeqOfVarSizeIA5StringFixedSizeAlias_BusCre/1  "<arr>"
  i16_SeqOfVarSizeOctetStringFixedSizeAlias_BusSel1/1 -> o16_SeqOfVarSizeOctetStringFixedSizeAlias_BusCre/1  "<arr>"
  i22_SeqOfVarSizeEnumAlias_BusSel1/1 -> o22_SeqOfVarSizeEnumAlias_BusCre/1  "<arr>"
